simulink model "Sim"  (R2025b)
settings: Solver=VariableStepAuto  StartTime=0.0  StopTime=simTime  RelTol=1e-3
values from neighbouring files (symbols this model uses):
  S1 = Tset + deadband    (= 22.8)    [Logic.m]
  S2 = Tset - deadband    (= 21.2)    [Logic.m]
  To = 32    [Logic.m]    (also in Logic2.m)
undefined symbols (not defined in the file or in its folder): k1, k2, k3

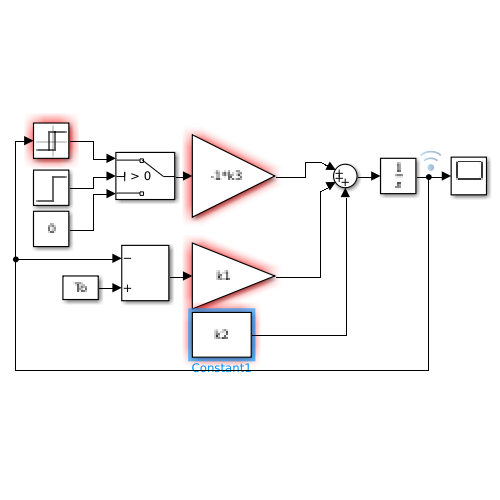
[thumbnail: Simulink's stored preview of the top-level diagram]
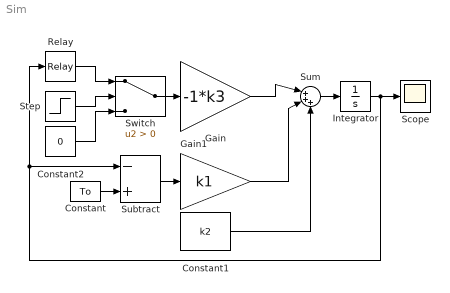
== system Sim ==
  Constant : Constant  Value=To
  Constant1 : Constant  Value=k2
  Constant2 : Constant  Value=0
  Gain : Gain  Gain=-1*k3
  Gain1 : Gain  Gain=k1
  Integrator : Integrator  InitialCondition=To
  Relay : Relay  OnSwitchValue=S1  OffSwitchValue=S2
  Scope : Scope
      settings: ActiveDisplayYMinimum=19.859457013277769  ActiveDisplayYMaximum=33.36370913517699
  Step : Step  Time=60  SampleTime=0
  Subtract : Sum  Inputs=-+
  Sum : Sum  Inputs=|+++
  Switch : Switch  Criteria=u2 > Threshold  SaturateOnIntegerOverflow=off  InputSameDT=off
  wires:
  Subtract/1 -> Gain1/1
  Constant/1 -> Subtract/2
  Gain/1 -> Sum/1
  Gain1/1 -> Sum/2
  Integrator/1 -> Scope/1, Subtract/1, Relay/1
  Sum/1 -> Integrator/1
  Constant1/1 -> Sum/3
  Step/1 -> Switch/2
  Switch/1 -> Gain/1
  Relay/1 -> Switch/1
  Constant2/1 -> Switch/3
